simulink subsystem "model_inductance_L2_sensitivity_distance"  (R2024a)
settings: Solver=VariableStepAuto  StartTime=0.0  StopTime=10.0  RelTol=1e-3
values from neighbouring files (symbols this model uses):
  d = 0.20    (= 0.2)    [maglev_parameters.m]
  r = 0.020    (= 0.02)    [maglev_parameters.m]
settings Model: Creator=Bocchio  LastModifiedBy=Bocchio

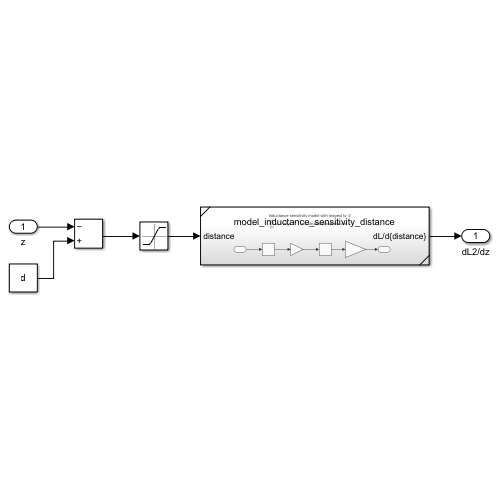
[thumbnail: Simulink's stored preview of the top-level diagram]
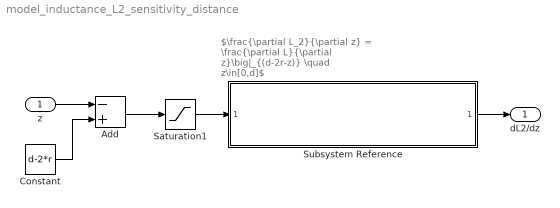
== system model_inductance_L2_sensitivity_distance ==
  note: $\frac{\partial L_2}{\partial z} = \frac{\partial L}{\partial z}\big|_{(d-2r-z)} \quad z\in[0,d]$
  z : Inport
  Add : Sum  Inputs=-+
  Constant : Constant  Value=d-2*r
  Saturation1 : Saturate  UpperLimit=d  LowerLimit=0
  Subsystem Reference : Subsystem  ReferencedSubsystem=model_inductance_sensitivity_distance
  dL2/dz : Outport
  wires:
  Subsystem Reference/1 -> dL2/dz/1
  Saturation1/1 -> Subsystem Reference/1
  Add/1 -> Saturation1/1
  Constant/1 -> Add/2
  z/1 -> Add/1
